simulink library "dlbsBlockSum"  (R2025b)
settings: Solver=VariableStepAuto  StartTime=0.0  StopTime=10.0  RelTol=1e-3
libraries: dlbsBlockExtractGradientGF x1, dlbsBlockInsertGradientGF x1
settings Model: Creator=lt6037  LastModifiedBy=lt6037

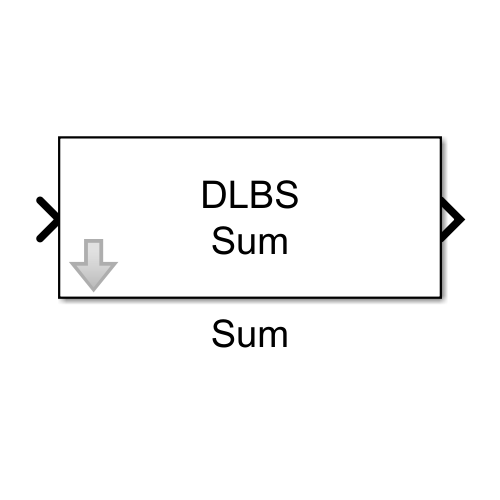
[thumbnail: Simulink's stored preview of the top-level diagram]
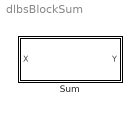
== system dlbsBlockSum ==
  Sum : Subsystem
      mask help: Computes the sum over all elements of an input tensor, producing a scalar output.
      mask Help: web("dlbsHelpBlockSum.html")
      mask Display: fprintf("DLBS\nSum")

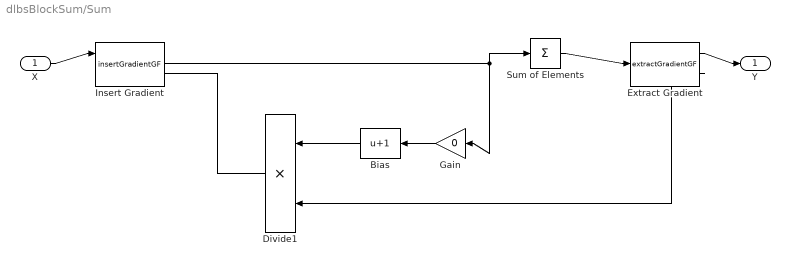
== system dlbsBlockSum/Sum ==
  X : Inport
  Bias : Bias  Bias=1  SaturateOnIntegerOverflow=off
  Divide1 : Product  Inputs=**
  Extract Gradient : dlbsBlockExtractGradientGF/extractGradientGF
  Gain : Gain  Gain=0
  Insert Gradient : dlbsBlockInsertGradientGF/insertGradientGF
  Sum of Elements : Sum  Inputs=+
  Y : Outport
  wires:
  Insert Gradient/1 -> Gain/1, Sum of Elements/1
  Gain/1 -> Bias/1
  Bias/1 -> Divide1/1
  Sum of Elements/1 -> Extract Gradient/1
  Divide1/1 -> Insert Gradient/2
  Extract Gradient/2 -> Divide1/2
  X/1 -> Insert Gradient/1
  Extract Gradient/1 -> Y/1
